simulink model "rtwdemo_sil_block"  (Simulink 7.6)
settings: Solver=ode3  StartTime=0.0  StopTime=10  FixedStep=0.01  RelTol=1e-3
PostLoadFcn:
  | overrides='{''SupportContinuousTime'',''SaveTime'',''SaveOutput'',''LaunchReport''}';
  | rtwconfiguredemo(gcs,'floating',false,overrides);
  | clear overrides
Description:
  | Software-in-the-Loop Code Verification
settings Model: Creator=The MathWorks Inc.  ExtModeAutoUpdateStatusClock=off
settings MATStruct: SampleTime=0.01  Offset=0  Priority=[20.0]
settings DataIOCC: LimitDataPoints=off  SignalLogging=off  ReturnWorkspaceOutputs=on  SignalLoggingName=sigsOut
settings OptimizationCC: InlineParams=on  UseIntDivNetSlope=on  InlineInvariantSignals=on  EnhancedBackFolding=on  BooleansAsBitfields=on  PassReuseOutputArgsAs=Individual arguments  StateBitsets=on  DataBitsets=on  UseTempVars=on  ZeroExternalMemoryAtStartup=off  ZeroInternalMemoryAtStartup=off  NoFixptDivByZeroProtection=on  EfficientFloat2IntCast=on  OptimizeModelRefInitCode=on  LifeSpan=1
settings DebuggingCC: UnderspecifiedInitializationDetection=Simplified  MergeDetectMultiDrivingBlocksExec=error  CheckExecutionContextPreStartOutputMsg=on  CheckExecutionContextRuntimeOutputMsg=on  SolverPrmCheckMsg=none  StrictBusMsg=ErrorOnBusTreatedAsVector
settings HardwareCC: ProdIntDivRoundTo=Zero  ProdEndianess=LittleEndian  ProdHWDeviceType=Specified  TargetEndianess=LittleEndian  TargetHWDeviceType=Generic->MATLAB Host Computer
settings RTWCC: SystemTargetFile=ert.tlc  TemplateMakefile=ert_default_tmf  Description=Real-Time Workshop Embedded Coder  GenerateReport=on  RTWVerbose=off  ProcessScript=ert_make_rtw_hook  IncludeHyperlinkInReport=on  GenerateTraceInfo=on  GenerateTraceReport=on  GenerateTraceReportSl=on  GenerateTraceReportSf=on  GenerateTraceReportEml=on
settings CodeAppCC: ForceParamTrailComments=on  IgnoreCustomStorageClasses=off  IgnoreTestpoints=on  SimulinkDataObjDesc=on  CustomSymbolStrGlobalVar=rt$N$M  CustomSymbolStrType=$N$M  CustomSymbolStrFcn=$N$M$F  CustomSymbolStrMacro=$N$M  InsertBlockDesc=on
settings ERTTargetCC: MultiwordLength=2048  GenerateSampleERTMain=on  IncludeMdlTerminateFcn=off  CombineSignalStateStructs=on  SupportNonFinite=off  SupportComplex=off  SupportContinuousTime=on  InlinedParameterPlacement=NonHierarchical  ERTCustomFileTemplate=example_file_process.tlc  ERTFilePackagingFormat=CompactWithDataFile  ConvertIfToSwitch=off

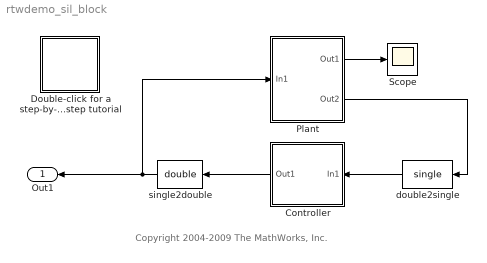
== system rtwdemo_sil_block ==
  note: Copyright 2004-2009 The MathWorks, Inc.
  Controller : Subsystem  TreatAsAtomicUnit=on
      settings: RTWFcnNameOpts=Use subsystem name  RTWFileNameOpts=Use function name
  Double-click for a step-by-step tutorial : Subsystem
      settings: OpenFcn=showdemo('rtwdemo_sil_pil_script');
      mask Type: Info
      mask Display: image(imread('targets_demo_info.bmp','bmp'),'center')
  Plant : Subsystem
  Scope : Scope
      settings: TimeRange=10  YMin=0  YMax=400
  double2single : DataTypeConversion  OutDataTypeStr=single
  single2double : DataTypeConversion  OutDataTypeStr=double
  Out1 : Outport
  wires:
  Plant/1(Out1) -> Scope/1
  Plant/2(Out2) -> double2single/1
  double2single/1 -> Controller/1(In1)
  single2double/1 -> Out1/1, Plant/1(In1)
  Controller/1(Out1) -> single2double/1

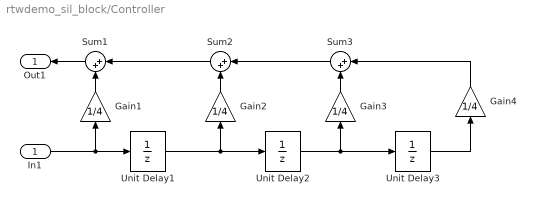
== system rtwdemo_sil_block/Controller ==
  In1 : Inport  SampleTime=.01
  Gain{1..4} (4 alike) : Gain  Gain=1/4  SaturateOnIntegerOverflow=on  ParamDataTypeStr=Inherit: Same as input
  Sum1 : Sum  Inputs=|++  SaturateOnIntegerOverflow=on  InputSameDT=on  OutDataTypeStr=Inherit: Same as first input
  Sum2 : Sum  Inputs=|++  SaturateOnIntegerOverflow=on  InputSameDT=on  OutDataTypeStr=Inherit: Same as first input
  Sum3 : Sum  Inputs=|++  SaturateOnIntegerOverflow=on  InputSameDT=on  OutDataTypeStr=Inherit: Same as first input
  Unit Delay1 : UnitDelay  SampleTime=-1
  Unit Delay2 : UnitDelay  SampleTime=-1
  Unit Delay3 : UnitDelay  SampleTime=-1
  Out1 : Outport
  wires:
  Gain1/1 -> Sum1/2
  In1/1 -> Unit Delay1/1, Gain1/1
  Sum1/1 -> Out1/1
  Sum3/1 -> Sum2/1
  Sum2/1 -> Sum1/1
  Unit Delay1/1 -> Unit Delay2/1, Gain2/1
  Unit Delay2/1 -> Unit Delay3/1, Gain3/1
  Unit Delay3/1 -> Gain4/1
  Gain4/1 -> Sum3/1
  Gain3/1 -> Sum3/2
  Gain2/1 -> Sum2/2

== system rtwdemo_sil_block/Double-click for a step-by-step tutorial ==

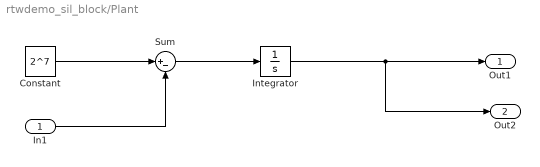
== system rtwdemo_sil_block/Plant ==
  In1 : Inport
  Constant : Constant  Value=2^7
  Integrator : Integrator
  Sum : Sum  Inputs=|+-  SaturateOnIntegerOverflow=on  InputSameDT=on  OutDataTypeStr=Inherit: Same as first input
  Out1 : Outport
  Out2 : Outport  Port=2
  wires:
  Integrator/1 -> Out1/1, Out2/1
  Sum/1 -> Integrator/1
  Constant/1 -> Sum/1
  In1/1 -> Sum/2
